simulink model "Counter"  (R2025b)
settings: Solver=FixedStepDiscrete  StartTime=0.0  StopTime=10.0  FixedStep=0.01  MaxStep=0.01  RelTol=1e-3
settings Model: Creator=soura  LastModifiedBy=soura

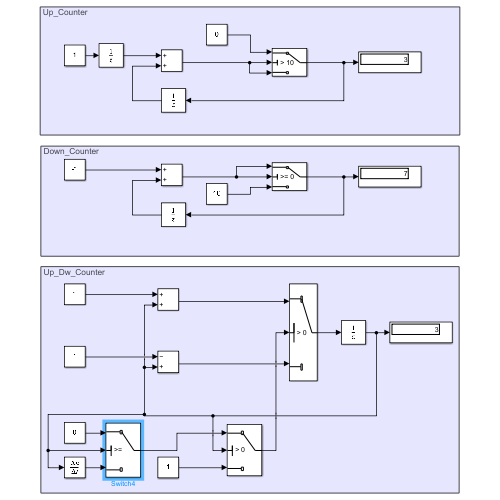
[thumbnail: Simulink's stored preview of the top-level diagram]
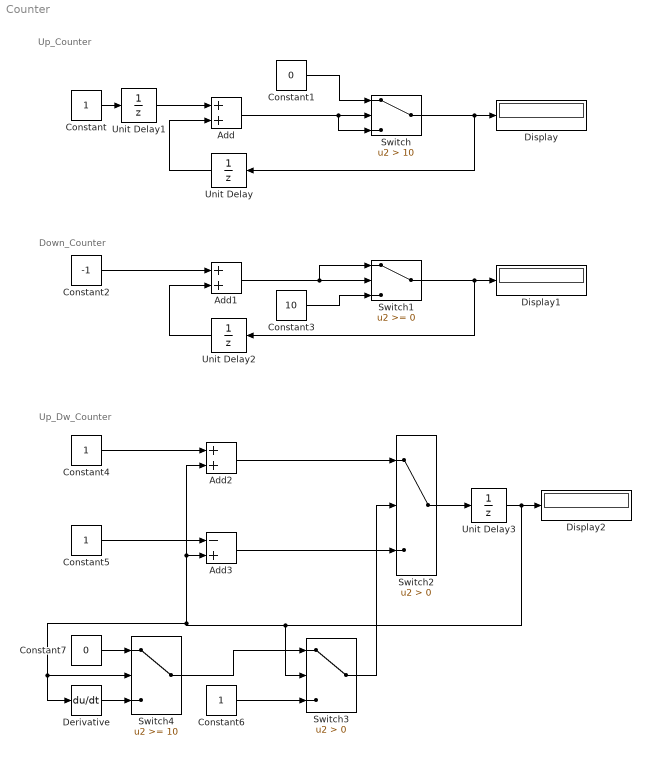
== system Counter ==
  note: Up_Dw_Counter
  note: Down_Counter
  note: Up_Counter
  Add : Sum
  Add1 : Sum
  Add2 : Sum
  Add3 : Sum  Inputs=-+
  Constant{,4..6} (4 alike) : Constant
  Constant1 : Constant  Value=0
  Constant2 : Constant  Value=-1
  Constant3 : Constant  Value=10
  Constant7 : Constant  Value=0
  Derivative : Derivative
  Display : Display
  Display1 : Display
  Display2 : Display
  Switch : Switch  Criteria=u2 > Threshold  Threshold=10  SaturateOnIntegerOverflow=off  InputSameDT=off
  Switch1 : Switch  SaturateOnIntegerOverflow=off  InputSameDT=off
  Switch2 : Switch  Criteria=u2 > Threshold  SaturateOnIntegerOverflow=off  InputSameDT=off
  Switch3 : Switch  Criteria=u2 > Threshold  SaturateOnIntegerOverflow=off  InputSameDT=off
  Switch4 : Switch  Threshold=10  SaturateOnIntegerOverflow=off  InputSameDT=off
  Unit Delay{,1..3} (4 alike) : UnitDelay  SampleTime=-1  HasFrameUpgradeWarning=on
  wires:
  Constant/1 -> Unit Delay1/1
  Unit Delay/1 -> Add/2
  Constant1/1 -> Switch/1
  Add/1 -> Switch/3, Switch/2
  Switch/1 -> Unit Delay/1, Display/1
  Unit Delay1/1 -> Add/1
  Constant2/1 -> Add1/1
  Switch1/1 -> Display1/1, Unit Delay2/1
  Add1/1 -> Switch1/1, Switch1/2
  Unit Delay2/1 -> Add1/2
  Constant3/1 -> Switch1/3
  Constant4/1 -> Add2/1
  Constant5/1 -> Add3/1
  Add2/1 -> Switch2/1
  Add3/1 -> Switch2/3
  Switch2/1 -> Unit Delay3/1
  Switch3/1 -> Switch2/2
  Unit Delay3/1 -> Display2/1, Switch3/2, Derivative/1, Switch4/2, Add3/2, Add2/2
  Switch4/1 -> Switch3/1
  Derivative/1 -> Switch4/3
  Constant7/1 -> Switch4/1
  Constant6/1 -> Switch3/3
